simulink model "rx2"  (R2022b)
settings: Solver=FixedStepDiscrete  StartTime=0.0  StopTime=3.3E6  FixedStep=1  RelTol=1e-3  EnableMultiTasking=on
model workspace (MAT data in the model file):
  mwTaskManagerKernelLatency = 0
undefined symbols (not defined in the file or in its folder): Add, jsin, magnitude, rom_pilot_conj_tt, Shift
libraries: hdlsllib x3231, whdlutilities x525, simulink x260, whdlmod x112, whdledac x26, dsphdlmathfun2 x24, commchan3 x1
(part 46 of 59)

== system rx2/demode1/chan_est1/Subsystem/HDL_DUT6/delta_estimator/iteration_estimation/register ==
  data_in : Inport
  valid_in : Inport  Port=2
  to_0 : Inport  Port=3
  Constant : Constant  OutDataTypeStr=fixdt(0,2,0)
  Ground : Ground
  Logical Operator : Logic  Operator=NOT  AllPortsSameDT=off  OutDataTypeStr=boolean
  Simple Dual Port RAM : hdlsllib/HDL RAMs/Simple Dual Port RAM  ram_size=2
  Switch : Switch  Criteria=u2 ~= 0  SaturateOnIntegerOverflow=off  InputSameDT=off
  data_out : Outport
  wires:
  data_in/1 -> Switch/1
  Simple Dual Port RAM/1 -> data_out/1
  Constant/1 -> Simple Dual Port RAM/4, Simple Dual Port RAM/2
  valid_in/1 -> Simple Dual Port RAM/3
  to_0/1 -> Logical Operator/1
  Logical Operator/1 -> Switch/2
  Ground/1 -> Switch/3
  Switch/1 -> Simple Dual Port RAM/1

== system rx2/demode1/chan_est1/Subsystem/HDL_DUT6/delta_estimator/iteration_estimation1/register ==
  data_in : Inport
  valid_in : Inport  Port=2
  to_0 : Inport  Port=3
  Constant : Constant  OutDataTypeStr=fixdt(0,2,0)
  Ground : Ground
  Logical Operator : Logic  Operator=NOT  AllPortsSameDT=off  OutDataTypeStr=boolean
  Simple Dual Port RAM : hdlsllib/HDL RAMs/Simple Dual Port RAM  ram_size=2
  Switch : Switch  Criteria=u2 ~= 0  SaturateOnIntegerOverflow=off  InputSameDT=off
  data_out : Outport
  wires:
  Switch/1 -> Simple Dual Port RAM/1
  Ground/1 -> Switch/3
  Logical Operator/1 -> Switch/2
  to_0/1 -> Logical Operator/1
  valid_in/1 -> Simple Dual Port RAM/3
  Constant/1 -> Simple Dual Port RAM/2, Simple Dual Port RAM/4
  Simple Dual Port RAM/1 -> data_out/1
  data_in/1 -> Switch/1

== system rx2/demode1/chan_est1/Subsystem/HDL_DUT7/delta_estimator/iteration_estimation/register ==
  data_in : Inport
  valid_in : Inport  Port=2
  to_0 : Inport  Port=3
  Constant : Constant  OutDataTypeStr=fixdt(0,2,0)
  Ground : Ground
  Logical Operator : Logic  Operator=NOT  AllPortsSameDT=off  OutDataTypeStr=boolean
  Simple Dual Port RAM : hdlsllib/HDL RAMs/Simple Dual Port RAM  ram_size=2
  Switch : Switch  Criteria=u2 ~= 0  SaturateOnIntegerOverflow=off  InputSameDT=off
  data_out : Outport
  wires:
  data_in/1 -> Switch/1
  Simple Dual Port RAM/1 -> data_out/1
  Constant/1 -> Simple Dual Port RAM/4, Simple Dual Port RAM/2
  valid_in/1 -> Simple Dual Port RAM/3
  to_0/1 -> Logical Operator/1
  Logical Operator/1 -> Switch/2
  Ground/1 -> Switch/3
  Switch/1 -> Simple Dual Port RAM/1

== system rx2/demode1/chan_est1/Subsystem/HDL_DUT7/delta_estimator/iteration_estimation1/register ==
  data_in : Inport
  valid_in : Inport  Port=2
  to_0 : Inport  Port=3
  Constant : Constant  OutDataTypeStr=fixdt(0,2,0)
  Ground : Ground
  Logical Operator : Logic  Operator=NOT  AllPortsSameDT=off  OutDataTypeStr=boolean
  Simple Dual Port RAM : hdlsllib/HDL RAMs/Simple Dual Port RAM  ram_size=2
  Switch : Switch  Criteria=u2 ~= 0  SaturateOnIntegerOverflow=off  InputSameDT=off
  data_out : Outport
  wires:
  Switch/1 -> Simple Dual Port RAM/1
  Ground/1 -> Switch/3
  Logical Operator/1 -> Switch/2
  to_0/1 -> Logical Operator/1
  valid_in/1 -> Simple Dual Port RAM/3
  Constant/1 -> Simple Dual Port RAM/2, Simple Dual Port RAM/4
  Simple Dual Port RAM/1 -> data_out/1
  data_in/1 -> Switch/1

== system rx2/process1/decoder/p-p/Subsystem2/Subsystem/Subsystem1/Subsystem ==
  data1 : Inport  OutDataTypeStr=data_type
  wr_addr : Inport  Port=2
  wr_en1 : Inport  Port=3
  rd_addr : Inport  Port=4
  Mux : Mux  Inputs=2
  Selector : Selector  InputPortWidth=8  IndexOptions=Index vector (dialog)  Indices=[1:4]  OutputSizes=1
  Selector1 : Selector  InputPortWidth=8  IndexOptions=Index vector (dialog)  Indices=[5:8]  OutputSizes=1
  Subsystem1 : Subsystem
  Subsystem4 : Subsystem
  rd_dout : Outport  PortDimensions=8  VectorParamsAs1DForOutWhenUnconnected=off
  wires:
  wr_addr/1 -> Subsystem1/2(wr_addr1), Subsystem4/2(wr_addr1)
  rd_addr/1 -> Subsystem1/4(rd_addr1), Subsystem4/4(rd_addr1)
  wr_en1/1 -> Subsystem1/3(wr_en2), Subsystem4/3(wr_en2)
  Mux/1 -> rd_dout/1
  Subsystem4/1(rd_dout1) -> Mux/1
  Subsystem1/1(rd_dout1) -> Mux/2
  data1/1 -> Selector1/1, Selector/1
  Selector/1 -> Subsystem4/1(data2)
  Selector1/1 -> Subsystem1/1(data2)

== system rx2/process1/decoder/p-p/Subsystem2/Subsystem/Subsystem1/Subsystem1 ==
  data1 : Inport  OutDataTypeStr=data_type
  wr_addr : Inport  Port=2
  wr_en1 : Inport  Port=3
  rd_addr : Inport  Port=4
  Mux : Mux  Inputs=2
  Selector : Selector  InputPortWidth=8  IndexOptions=Index vector (dialog)  Indices=[1:4]  OutputSizes=1
  Selector1 : Selector  InputPortWidth=8  IndexOptions=Index vector (dialog)  Indices=[5:8]  OutputSizes=1
  Subsystem1 : Subsystem
  Subsystem4 : Subsystem
  rd_dout : Outport  PortDimensions=8  VectorParamsAs1DForOutWhenUnconnected=off
  wires:
  Selector1/1 -> Subsystem1/1(data2)
  Selector/1 -> Subsystem4/1(data2)
  data1/1 -> Selector/1, Selector1/1
  Subsystem1/1(rd_dout1) -> Mux/2
  Subsystem4/1(rd_dout1) -> Mux/1
  Mux/1 -> rd_dout/1
  wr_en1/1 -> Subsystem1/3(wr_en2), Subsystem4/3(wr_en2)
  rd_addr/1 -> Subsystem1/4(rd_addr1), Subsystem4/4(rd_addr1)
  wr_addr/1 -> Subsystem1/2(wr_addr1), Subsystem4/2(wr_addr1)

== system rx2/process1/decoder/p-p/Subsystem2/Subsystem/Subsystem2/Subsystem ==
  data1 : Inport  OutDataTypeStr=data_type
  wr_addr : Inport  Port=2
  wr_en1 : Inport  Port=3
  rd_addr : Inport  Port=4
  Mux : Mux  Inputs=2
  Selector : Selector  InputPortWidth=8  IndexOptions=Index vector (dialog)  Indices=[1:4]  OutputSizes=1
  Selector1 : Selector  InputPortWidth=8  IndexOptions=Index vector (dialog)  Indices=[5:8]  OutputSizes=1
  Subsystem1 : Subsystem
  Subsystem4 : Subsystem
  rd_dout : Outport  PortDimensions=8  VectorParamsAs1DForOutWhenUnconnected=off
  wires:
  wr_addr/1 -> Subsystem1/2(wr_addr1), Subsystem4/2(wr_addr1)
  rd_addr/1 -> Subsystem1/4(rd_addr1), Subsystem4/4(rd_addr1)
  wr_en1/1 -> Subsystem1/3(wr_en2), Subsystem4/3(wr_en2)
  Mux/1 -> rd_dout/1
  Subsystem4/1(rd_dout1) -> Mux/1
  Subsystem1/1(rd_dout1) -> Mux/2
  data1/1 -> Selector1/1, Selector/1
  Selector/1 -> Subsystem4/1(data2)
  Selector1/1 -> Subsystem1/1(data2)

== system rx2/process1/decoder/p-p/Subsystem2/Subsystem/Subsystem2/Subsystem1 ==
  data1 : Inport  OutDataTypeStr=data_type
  wr_addr : Inport  Port=2
  wr_en1 : Inport  Port=3
  rd_addr : Inport  Port=4
  Mux : Mux  Inputs=2
  Selector : Selector  InputPortWidth=8  IndexOptions=Index vector (dialog)  Indices=[1:4]  OutputSizes=1
  Selector1 : Selector  InputPortWidth=8  IndexOptions=Index vector (dialog)  Indices=[5:8]  OutputSizes=1
  Subsystem1 : Subsystem
  Subsystem4 : Subsystem
  rd_dout : Outport  PortDimensions=8  VectorParamsAs1DForOutWhenUnconnected=off
  wires:
  Selector1/1 -> Subsystem1/1(data2)
  Selector/1 -> Subsystem4/1(data2)
  data1/1 -> Selector/1, Selector1/1
  Subsystem1/1(rd_dout1) -> Mux/2
  Subsystem4/1(rd_dout1) -> Mux/1
  Mux/1 -> rd_dout/1
  wr_en1/1 -> Subsystem1/3(wr_en2), Subsystem4/3(wr_en2)
  rd_addr/1 -> Subsystem1/4(rd_addr1), Subsystem4/4(rd_addr1)
  wr_addr/1 -> Subsystem1/2(wr_addr1), Subsystem4/2(wr_addr1)

== system rx2/process1/decoder/p-p/Subsystem2/Subsystem1/Subsystem1/Subsystem ==
  data1 : Inport  OutDataTypeStr=data_type
  wr_addr : Inport  Port=2
  wr_en1 : Inport  Port=3
  rd_addr : Inport  Port=4
  Mux : Mux  Inputs=2
  Selector : Selector  InputPortWidth=8  IndexOptions=Index vector (dialog)  Indices=[1:4]  OutputSizes=1
  Selector1 : Selector  InputPortWidth=8  IndexOptions=Index vector (dialog)  Indices=[5:8]  OutputSizes=1
  Subsystem1 : Subsystem
  Subsystem4 : Subsystem
  rd_dout : Outport  PortDimensions=8  VectorParamsAs1DForOutWhenUnconnected=off
  wires:
  wr_addr/1 -> Subsystem1/2(wr_addr1), Subsystem4/2(wr_addr1)
  rd_addr/1 -> Subsystem1/4(rd_addr1), Subsystem4/4(rd_addr1)
  wr_en1/1 -> Subsystem1/3(wr_en2), Subsystem4/3(wr_en2)
  Mux/1 -> rd_dout/1
  Subsystem4/1(rd_dout1) -> Mux/1
  Subsystem1/1(rd_dout1) -> Mux/2
  data1/1 -> Selector1/1, Selector/1
  Selector/1 -> Subsystem4/1(data2)
  Selector1/1 -> Subsystem1/1(data2)

== system rx2/process1/decoder/p-p/Subsystem2/Subsystem1/Subsystem1/Subsystem1 ==
  data1 : Inport  OutDataTypeStr=data_type
  wr_addr : Inport  Port=2
  wr_en1 : Inport  Port=3
  rd_addr : Inport  Port=4
  Mux : Mux  Inputs=2
  Selector : Selector  InputPortWidth=8  IndexOptions=Index vector (dialog)  Indices=[1:4]  OutputSizes=1
  Selector1 : Selector  InputPortWidth=8  IndexOptions=Index vector (dialog)  Indices=[5:8]  OutputSizes=1
  Subsystem1 : Subsystem
  Subsystem4 : Subsystem
  rd_dout : Outport  PortDimensions=8  VectorParamsAs1DForOutWhenUnconnected=off
  wires:
  Selector1/1 -> Subsystem1/1(data2)
  Selector/1 -> Subsystem4/1(data2)
  data1/1 -> Selector/1, Selector1/1
  Subsystem1/1(rd_dout1) -> Mux/2
  Subsystem4/1(rd_dout1) -> Mux/1
  Mux/1 -> rd_dout/1
  wr_en1/1 -> Subsystem1/3(wr_en2), Subsystem4/3(wr_en2)
  rd_addr/1 -> Subsystem1/4(rd_addr1), Subsystem4/4(rd_addr1)
  wr_addr/1 -> Subsystem1/2(wr_addr1), Subsystem4/2(wr_addr1)

== system rx2/process1/decoder/p-p/Subsystem2/Subsystem1/Subsystem2/Subsystem ==
  data1 : Inport  OutDataTypeStr=data_type
  wr_addr : Inport  Port=2
  wr_en1 : Inport  Port=3
  rd_addr : Inport  Port=4
  Mux : Mux  Inputs=2
  Selector : Selector  InputPortWidth=8  IndexOptions=Index vector (dialog)  Indices=[1:4]  OutputSizes=1
  Selector1 : Selector  InputPortWidth=8  IndexOptions=Index vector (dialog)  Indices=[5:8]  OutputSizes=1
  Subsystem1 : Subsystem
  Subsystem4 : Subsystem
  rd_dout : Outport  PortDimensions=8  VectorParamsAs1DForOutWhenUnconnected=off
  wires:
  wr_addr/1 -> Subsystem1/2(wr_addr1), Subsystem4/2(wr_addr1)
  rd_addr/1 -> Subsystem1/4(rd_addr1), Subsystem4/4(rd_addr1)
  wr_en1/1 -> Subsystem1/3(wr_en2), Subsystem4/3(wr_en2)
  Mux/1 -> rd_dout/1
  Subsystem4/1(rd_dout1) -> Mux/1
  Subsystem1/1(rd_dout1) -> Mux/2
  data1/1 -> Selector1/1, Selector/1
  Selector/1 -> Subsystem4/1(data2)
  Selector1/1 -> Subsystem1/1(data2)

== system rx2/process1/decoder/p-p/Subsystem2/Subsystem1/Subsystem2/Subsystem1 ==
  data1 : Inport  OutDataTypeStr=data_type
  wr_addr : Inport  Port=2
  wr_en1 : Inport  Port=3
  rd_addr : Inport  Port=4
  Mux : Mux  Inputs=2
  Selector : Selector  InputPortWidth=8  IndexOptions=Index vector (dialog)  Indices=[1:4]  OutputSizes=1
  Selector1 : Selector  InputPortWidth=8  IndexOptions=Index vector (dialog)  Indices=[5:8]  OutputSizes=1
  Subsystem1 : Subsystem
  Subsystem4 : Subsystem
  rd_dout : Outport  PortDimensions=8  VectorParamsAs1DForOutWhenUnconnected=off
  wires:
  Selector1/1 -> Subsystem1/1(data2)
  Selector/1 -> Subsystem4/1(data2)
  data1/1 -> Selector/1, Selector1/1
  Subsystem1/1(rd_dout1) -> Mux/2
  Subsystem4/1(rd_dout1) -> Mux/1
  Mux/1 -> rd_dout/1
  wr_en1/1 -> Subsystem1/3(wr_en2), Subsystem4/3(wr_en2)
  rd_addr/1 -> Subsystem1/4(rd_addr1), Subsystem4/4(rd_addr1)
  wr_addr/1 -> Subsystem1/2(wr_addr1), Subsystem4/2(wr_addr1)

== system rx2/process10/decoder/p-p/Subsystem2/Subsystem/Subsystem1/Subsystem ==
  data1 : Inport  OutDataTypeStr=data_type
  wr_addr : Inport  Port=2
  wr_en1 : Inport  Port=3
  rd_addr : Inport  Port=4
  Mux : Mux  Inputs=2
  Selector : Selector  InputPortWidth=8  IndexOptions=Index vector (dialog)  Indices=[1:4]  OutputSizes=1
  Selector1 : Selector  InputPortWidth=8  IndexOptions=Index vector (dialog)  Indices=[5:8]  OutputSizes=1
  Subsystem1 : Subsystem
  Subsystem4 : Subsystem
  rd_dout : Outport  PortDimensions=8  VectorParamsAs1DForOutWhenUnconnected=off
  wires:
  wr_addr/1 -> Subsystem1/2(wr_addr1), Subsystem4/2(wr_addr1)
  rd_addr/1 -> Subsystem1/4(rd_addr1), Subsystem4/4(rd_addr1)
  wr_en1/1 -> Subsystem1/3(wr_en2), Subsystem4/3(wr_en2)
  Mux/1 -> rd_dout/1
  Subsystem4/1(rd_dout1) -> Mux/1
  Subsystem1/1(rd_dout1) -> Mux/2
  data1/1 -> Selector1/1, Selector/1
  Selector/1 -> Subsystem4/1(data2)
  Selector1/1 -> Subsystem1/1(data2)

== system rx2/process10/decoder/p-p/Subsystem2/Subsystem/Subsystem1/Subsystem1 ==
  data1 : Inport  OutDataTypeStr=data_type
  wr_addr : Inport  Port=2
  wr_en1 : Inport  Port=3
  rd_addr : Inport  Port=4
  Mux : Mux  Inputs=2
  Selector : Selector  InputPortWidth=8  IndexOptions=Index vector (dialog)  Indices=[1:4]  OutputSizes=1
  Selector1 : Selector  InputPortWidth=8  IndexOptions=Index vector (dialog)  Indices=[5:8]  OutputSizes=1
  Subsystem1 : Subsystem
  Subsystem4 : Subsystem
  rd_dout : Outport  PortDimensions=8  VectorParamsAs1DForOutWhenUnconnected=off
  wires:
  Selector1/1 -> Subsystem1/1(data2)
  Selector/1 -> Subsystem4/1(data2)
  data1/1 -> Selector/1, Selector1/1
  Subsystem1/1(rd_dout1) -> Mux/2
  Subsystem4/1(rd_dout1) -> Mux/1
  Mux/1 -> rd_dout/1
  wr_en1/1 -> Subsystem1/3(wr_en2), Subsystem4/3(wr_en2)
  rd_addr/1 -> Subsystem1/4(rd_addr1), Subsystem4/4(rd_addr1)
  wr_addr/1 -> Subsystem1/2(wr_addr1), Subsystem4/2(wr_addr1)

== system rx2/process10/decoder/p-p/Subsystem2/Subsystem/Subsystem2/Subsystem ==
  data1 : Inport  OutDataTypeStr=data_type
  wr_addr : Inport  Port=2
  wr_en1 : Inport  Port=3
  rd_addr : Inport  Port=4
  Mux : Mux  Inputs=2
  Selector : Selector  InputPortWidth=8  IndexOptions=Index vector (dialog)  Indices=[1:4]  OutputSizes=1
  Selector1 : Selector  InputPortWidth=8  IndexOptions=Index vector (dialog)  Indices=[5:8]  OutputSizes=1
  Subsystem1 : Subsystem
  Subsystem4 : Subsystem
  rd_dout : Outport  PortDimensions=8  VectorParamsAs1DForOutWhenUnconnected=off
  wires:
  wr_addr/1 -> Subsystem1/2(wr_addr1), Subsystem4/2(wr_addr1)
  rd_addr/1 -> Subsystem1/4(rd_addr1), Subsystem4/4(rd_addr1)
  wr_en1/1 -> Subsystem1/3(wr_en2), Subsystem4/3(wr_en2)
  Mux/1 -> rd_dout/1
  Subsystem4/1(rd_dout1) -> Mux/1
  Subsystem1/1(rd_dout1) -> Mux/2
  data1/1 -> Selector1/1, Selector/1
  Selector/1 -> Subsystem4/1(data2)
  Selector1/1 -> Subsystem1/1(data2)

== system rx2/process10/decoder/p-p/Subsystem2/Subsystem/Subsystem2/Subsystem1 ==
  data1 : Inport  OutDataTypeStr=data_type
  wr_addr : Inport  Port=2
  wr_en1 : Inport  Port=3
  rd_addr : Inport  Port=4
  Mux : Mux  Inputs=2
  Selector : Selector  InputPortWidth=8  IndexOptions=Index vector (dialog)  Indices=[1:4]  OutputSizes=1
  Selector1 : Selector  InputPortWidth=8  IndexOptions=Index vector (dialog)  Indices=[5:8]  OutputSizes=1
  Subsystem1 : Subsystem
  Subsystem4 : Subsystem
  rd_dout : Outport  PortDimensions=8  VectorParamsAs1DForOutWhenUnconnected=off
  wires:
  Selector1/1 -> Subsystem1/1(data2)
  Selector/1 -> Subsystem4/1(data2)
  data1/1 -> Selector/1, Selector1/1
  Subsystem1/1(rd_dout1) -> Mux/2
  Subsystem4/1(rd_dout1) -> Mux/1
  Mux/1 -> rd_dout/1
  wr_en1/1 -> Subsystem1/3(wr_en2), Subsystem4/3(wr_en2)
  rd_addr/1 -> Subsystem1/4(rd_addr1), Subsystem4/4(rd_addr1)
  wr_addr/1 -> Subsystem1/2(wr_addr1), Subsystem4/2(wr_addr1)

== system rx2/process10/decoder/p-p/Subsystem2/Subsystem1/Subsystem1/Subsystem ==
  data1 : Inport  OutDataTypeStr=data_type
  wr_addr : Inport  Port=2
  wr_en1 : Inport  Port=3
  rd_addr : Inport  Port=4
  Mux : Mux  Inputs=2
  Selector : Selector  InputPortWidth=8  IndexOptions=Index vector (dialog)  Indices=[1:4]  OutputSizes=1
  Selector1 : Selector  InputPortWidth=8  IndexOptions=Index vector (dialog)  Indices=[5:8]  OutputSizes=1
  Subsystem1 : Subsystem
  Subsystem4 : Subsystem
  rd_dout : Outport  PortDimensions=8  VectorParamsAs1DForOutWhenUnconnected=off
  wires:
  wr_addr/1 -> Subsystem1/2(wr_addr1), Subsystem4/2(wr_addr1)
  rd_addr/1 -> Subsystem1/4(rd_addr1), Subsystem4/4(rd_addr1)
  wr_en1/1 -> Subsystem1/3(wr_en2), Subsystem4/3(wr_en2)
  Mux/1 -> rd_dout/1
  Subsystem4/1(rd_dout1) -> Mux/1
  Subsystem1/1(rd_dout1) -> Mux/2
  data1/1 -> Selector1/1, Selector/1
  Selector/1 -> Subsystem4/1(data2)
  Selector1/1 -> Subsystem1/1(data2)

== system rx2/process10/decoder/p-p/Subsystem2/Subsystem1/Subsystem1/Subsystem1 ==
  data1 : Inport  OutDataTypeStr=data_type
  wr_addr : Inport  Port=2
  wr_en1 : Inport  Port=3
  rd_addr : Inport  Port=4
  Mux : Mux  Inputs=2
  Selector : Selector  InputPortWidth=8  IndexOptions=Index vector (dialog)  Indices=[1:4]  OutputSizes=1
  Selector1 : Selector  InputPortWidth=8  IndexOptions=Index vector (dialog)  Indices=[5:8]  OutputSizes=1
  Subsystem1 : Subsystem
  Subsystem4 : Subsystem
  rd_dout : Outport  PortDimensions=8  VectorParamsAs1DForOutWhenUnconnected=off
  wires:
  Selector1/1 -> Subsystem1/1(data2)
  Selector/1 -> Subsystem4/1(data2)
  data1/1 -> Selector/1, Selector1/1
  Subsystem1/1(rd_dout1) -> Mux/2
  Subsystem4/1(rd_dout1) -> Mux/1
  Mux/1 -> rd_dout/1
  wr_en1/1 -> Subsystem1/3(wr_en2), Subsystem4/3(wr_en2)
  rd_addr/1 -> Subsystem1/4(rd_addr1), Subsystem4/4(rd_addr1)
  wr_addr/1 -> Subsystem1/2(wr_addr1), Subsystem4/2(wr_addr1)

== system rx2/process10/decoder/p-p/Subsystem2/Subsystem1/Subsystem2/Subsystem ==
  data1 : Inport  OutDataTypeStr=data_type
  wr_addr : Inport  Port=2
  wr_en1 : Inport  Port=3
  rd_addr : Inport  Port=4
  Mux : Mux  Inputs=2
  Selector : Selector  InputPortWidth=8  IndexOptions=Index vector (dialog)  Indices=[1:4]  OutputSizes=1
  Selector1 : Selector  InputPortWidth=8  IndexOptions=Index vector (dialog)  Indices=[5:8]  OutputSizes=1
  Subsystem1 : Subsystem
  Subsystem4 : Subsystem
  rd_dout : Outport  PortDimensions=8  VectorParamsAs1DForOutWhenUnconnected=off
  wires:
  wr_addr/1 -> Subsystem1/2(wr_addr1), Subsystem4/2(wr_addr1)
  rd_addr/1 -> Subsystem1/4(rd_addr1), Subsystem4/4(rd_addr1)
  wr_en1/1 -> Subsystem1/3(wr_en2), Subsystem4/3(wr_en2)
  Mux/1 -> rd_dout/1
  Subsystem4/1(rd_dout1) -> Mux/1
  Subsystem1/1(rd_dout1) -> Mux/2
  data1/1 -> Selector1/1, Selector/1
  Selector/1 -> Subsystem4/1(data2)
  Selector1/1 -> Subsystem1/1(data2)

== system rx2/process10/decoder/p-p/Subsystem2/Subsystem1/Subsystem2/Subsystem1 ==
  data1 : Inport  OutDataTypeStr=data_type
  wr_addr : Inport  Port=2
  wr_en1 : Inport  Port=3
  rd_addr : Inport  Port=4
  Mux : Mux  Inputs=2
  Selector : Selector  InputPortWidth=8  IndexOptions=Index vector (dialog)  Indices=[1:4]  OutputSizes=1
  Selector1 : Selector  InputPortWidth=8  IndexOptions=Index vector (dialog)  Indices=[5:8]  OutputSizes=1
  Subsystem1 : Subsystem
  Subsystem4 : Subsystem
  rd_dout : Outport  PortDimensions=8  VectorParamsAs1DForOutWhenUnconnected=off
  wires:
  Selector1/1 -> Subsystem1/1(data2)
  Selector/1 -> Subsystem4/1(data2)
  data1/1 -> Selector/1, Selector1/1
  Subsystem1/1(rd_dout1) -> Mux/2
  Subsystem4/1(rd_dout1) -> Mux/1
  Mux/1 -> rd_dout/1
  wr_en1/1 -> Subsystem1/3(wr_en2), Subsystem4/3(wr_en2)
  rd_addr/1 -> Subsystem1/4(rd_addr1), Subsystem4/4(rd_addr1)
  wr_addr/1 -> Subsystem1/2(wr_addr1), Subsystem4/2(wr_addr1)

== system rx2/process11/decoder/p-p/Subsystem2/Subsystem/Subsystem1/Subsystem ==
  data1 : Inport  OutDataTypeStr=data_type
  wr_addr : Inport  Port=2
  wr_en1 : Inport  Port=3
  rd_addr : Inport  Port=4
  Mux : Mux  Inputs=2
  Selector : Selector  InputPortWidth=8  IndexOptions=Index vector (dialog)  Indices=[1:4]  OutputSizes=1
  Selector1 : Selector  InputPortWidth=8  IndexOptions=Index vector (dialog)  Indices=[5:8]  OutputSizes=1
  Subsystem1 : Subsystem
  Subsystem4 : Subsystem
  rd_dout : Outport  PortDimensions=8  VectorParamsAs1DForOutWhenUnconnected=off
  wires:
  Selector1/1 -> Subsystem1/1(data2)
  Selector/1 -> Subsystem4/1(data2)
  data1/1 -> Selector/1, Selector1/1
  Subsystem1/1(rd_dout1) -> Mux/2
  Subsystem4/1(rd_dout1) -> Mux/1
  Mux/1 -> rd_dout/1
  wr_en1/1 -> Subsystem4/3(wr_en2), Subsystem1/3(wr_en2)
  rd_addr/1 -> Subsystem4/4(rd_addr1), Subsystem1/4(rd_addr1)
  wr_addr/1 -> Subsystem4/2(wr_addr1), Subsystem1/2(wr_addr1)

== system rx2/process11/decoder/p-p/Subsystem2/Subsystem/Subsystem1/Subsystem1 ==
  data1 : Inport  OutDataTypeStr=data_type
  wr_addr : Inport  Port=2
  wr_en1 : Inport  Port=3
  rd_addr : Inport  Port=4
  Mux : Mux  Inputs=2
  Selector : Selector  InputPortWidth=8  IndexOptions=Index vector (dialog)  Indices=[1:4]  OutputSizes=1
  Selector1 : Selector  InputPortWidth=8  IndexOptions=Index vector (dialog)  Indices=[5:8]  OutputSizes=1
  Subsystem1 : Subsystem
  Subsystem4 : Subsystem
  rd_dout : Outport  PortDimensions=8  VectorParamsAs1DForOutWhenUnconnected=off
  wires:
  wr_addr/1 -> Subsystem4/2(wr_addr1), Subsystem1/2(wr_addr1)
  rd_addr/1 -> Subsystem4/4(rd_addr1), Subsystem1/4(rd_addr1)
  wr_en1/1 -> Subsystem4/3(wr_en2), Subsystem1/3(wr_en2)
  Mux/1 -> rd_dout/1
  Subsystem4/1(rd_dout1) -> Mux/1
  Subsystem1/1(rd_dout1) -> Mux/2
  data1/1 -> Selector1/1, Selector/1
  Selector/1 -> Subsystem4/1(data2)
  Selector1/1 -> Subsystem1/1(data2)

== system rx2/process11/decoder/p-p/Subsystem2/Subsystem/Subsystem2/Subsystem ==
  data1 : Inport  OutDataTypeStr=data_type
  wr_addr : Inport  Port=2
  wr_en1 : Inport  Port=3
  rd_addr : Inport  Port=4
  Mux : Mux  Inputs=2
  Selector : Selector  InputPortWidth=8  IndexOptions=Index vector (dialog)  Indices=[1:4]  OutputSizes=1
  Selector1 : Selector  InputPortWidth=8  IndexOptions=Index vector (dialog)  Indices=[5:8]  OutputSizes=1
  Subsystem1 : Subsystem
  Subsystem4 : Subsystem
  rd_dout : Outport  PortDimensions=8  VectorParamsAs1DForOutWhenUnconnected=off
  wires:
  Selector1/1 -> Subsystem1/1(data2)
  Selector/1 -> Subsystem4/1(data2)
  data1/1 -> Selector/1, Selector1/1
  Subsystem1/1(rd_dout1) -> Mux/2
  Subsystem4/1(rd_dout1) -> Mux/1
  Mux/1 -> rd_dout/1
  wr_en1/1 -> Subsystem4/3(wr_en2), Subsystem1/3(wr_en2)
  rd_addr/1 -> Subsystem4/4(rd_addr1), Subsystem1/4(rd_addr1)
  wr_addr/1 -> Subsystem4/2(wr_addr1), Subsystem1/2(wr_addr1)

== system rx2/process11/decoder/p-p/Subsystem2/Subsystem/Subsystem2/Subsystem1 ==
  data1 : Inport  OutDataTypeStr=data_type
  wr_addr : Inport  Port=2
  wr_en1 : Inport  Port=3
  rd_addr : Inport  Port=4
  Mux : Mux  Inputs=2
  Selector : Selector  InputPortWidth=8  IndexOptions=Index vector (dialog)  Indices=[1:4]  OutputSizes=1
  Selector1 : Selector  InputPortWidth=8  IndexOptions=Index vector (dialog)  Indices=[5:8]  OutputSizes=1
  Subsystem1 : Subsystem
  Subsystem4 : Subsystem
  rd_dout : Outport  PortDimensions=8  VectorParamsAs1DForOutWhenUnconnected=off
  wires:
  wr_addr/1 -> Subsystem4/2(wr_addr1), Subsystem1/2(wr_addr1)
  rd_addr/1 -> Subsystem4/4(rd_addr1), Subsystem1/4(rd_addr1)
  wr_en1/1 -> Subsystem4/3(wr_en2), Subsystem1/3(wr_en2)
  Mux/1 -> rd_dout/1
  Subsystem4/1(rd_dout1) -> Mux/1
  Subsystem1/1(rd_dout1) -> Mux/2
  data1/1 -> Selector1/1, Selector/1
  Selector/1 -> Subsystem4/1(data2)
  Selector1/1 -> Subsystem1/1(data2)

== system rx2/process11/decoder/p-p/Subsystem2/Subsystem1/Subsystem1/Subsystem ==
  data1 : Inport  OutDataTypeStr=data_type
  wr_addr : Inport  Port=2
  wr_en1 : Inport  Port=3
  rd_addr : Inport  Port=4
  Mux : Mux  Inputs=2
  Selector : Selector  InputPortWidth=8  IndexOptions=Index vector (dialog)  Indices=[1:4]  OutputSizes=1
  Selector1 : Selector  InputPortWidth=8  IndexOptions=Index vector (dialog)  Indices=[5:8]  OutputSizes=1
  Subsystem1 : Subsystem
  Subsystem4 : Subsystem
  rd_dout : Outport  PortDimensions=8  VectorParamsAs1DForOutWhenUnconnected=off
  wires:
  Selector1/1 -> Subsystem1/1(data2)
  Selector/1 -> Subsystem4/1(data2)
  data1/1 -> Selector/1, Selector1/1
  Subsystem1/1(rd_dout1) -> Mux/2
  Subsystem4/1(rd_dout1) -> Mux/1
  Mux/1 -> rd_dout/1
  wr_en1/1 -> Subsystem4/3(wr_en2), Subsystem1/3(wr_en2)
  rd_addr/1 -> Subsystem4/4(rd_addr1), Subsystem1/4(rd_addr1)
  wr_addr/1 -> Subsystem4/2(wr_addr1), Subsystem1/2(wr_addr1)

== system rx2/process11/decoder/p-p/Subsystem2/Subsystem1/Subsystem1/Subsystem1 ==
  data1 : Inport  OutDataTypeStr=data_type
  wr_addr : Inport  Port=2
  wr_en1 : Inport  Port=3
  rd_addr : Inport  Port=4
  Mux : Mux  Inputs=2
  Selector : Selector  InputPortWidth=8  IndexOptions=Index vector (dialog)  Indices=[1:4]  OutputSizes=1
  Selector1 : Selector  InputPortWidth=8  IndexOptions=Index vector (dialog)  Indices=[5:8]  OutputSizes=1
  Subsystem1 : Subsystem
  Subsystem4 : Subsystem
  rd_dout : Outport  PortDimensions=8  VectorParamsAs1DForOutWhenUnconnected=off
  wires:
  wr_addr/1 -> Subsystem4/2(wr_addr1), Subsystem1/2(wr_addr1)
  rd_addr/1 -> Subsystem4/4(rd_addr1), Subsystem1/4(rd_addr1)
  wr_en1/1 -> Subsystem4/3(wr_en2), Subsystem1/3(wr_en2)
  Mux/1 -> rd_dout/1
  Subsystem4/1(rd_dout1) -> Mux/1
  Subsystem1/1(rd_dout1) -> Mux/2
  data1/1 -> Selector1/1, Selector/1
  Selector/1 -> Subsystem4/1(data2)
  Selector1/1 -> Subsystem1/1(data2)

== system rx2/process11/decoder/p-p/Subsystem2/Subsystem1/Subsystem2/Subsystem ==
  data1 : Inport  OutDataTypeStr=data_type
  wr_addr : Inport  Port=2
  wr_en1 : Inport  Port=3
  rd_addr : Inport  Port=4
  Mux : Mux  Inputs=2
  Selector : Selector  InputPortWidth=8  IndexOptions=Index vector (dialog)  Indices=[1:4]  OutputSizes=1
  Selector1 : Selector  InputPortWidth=8  IndexOptions=Index vector (dialog)  Indices=[5:8]  OutputSizes=1
  Subsystem1 : Subsystem
  Subsystem4 : Subsystem
  rd_dout : Outport  PortDimensions=8  VectorParamsAs1DForOutWhenUnconnected=off
  wires:
  Selector1/1 -> Subsystem1/1(data2)
  Selector/1 -> Subsystem4/1(data2)
  data1/1 -> Selector/1, Selector1/1
  Subsystem1/1(rd_dout1) -> Mux/2
  Subsystem4/1(rd_dout1) -> Mux/1
  Mux/1 -> rd_dout/1
  wr_en1/1 -> Subsystem4/3(wr_en2), Subsystem1/3(wr_en2)
  rd_addr/1 -> Subsystem4/4(rd_addr1), Subsystem1/4(rd_addr1)
  wr_addr/1 -> Subsystem4/2(wr_addr1), Subsystem1/2(wr_addr1)

== system rx2/process11/decoder/p-p/Subsystem2/Subsystem1/Subsystem2/Subsystem1 ==
  data1 : Inport  OutDataTypeStr=data_type
  wr_addr : Inport  Port=2
  wr_en1 : Inport  Port=3
  rd_addr : Inport  Port=4
  Mux : Mux  Inputs=2
  Selector : Selector  InputPortWidth=8  IndexOptions=Index vector (dialog)  Indices=[1:4]  OutputSizes=1
  Selector1 : Selector  InputPortWidth=8  IndexOptions=Index vector (dialog)  Indices=[5:8]  OutputSizes=1
  Subsystem1 : Subsystem
  Subsystem4 : Subsystem
  rd_dout : Outport  PortDimensions=8  VectorParamsAs1DForOutWhenUnconnected=off
  wires:
  wr_addr/1 -> Subsystem4/2(wr_addr1), Subsystem1/2(wr_addr1)
  rd_addr/1 -> Subsystem4/4(rd_addr1), Subsystem1/4(rd_addr1)
  wr_en1/1 -> Subsystem4/3(wr_en2), Subsystem1/3(wr_en2)
  Mux/1 -> rd_dout/1
  Subsystem4/1(rd_dout1) -> Mux/1
  Subsystem1/1(rd_dout1) -> Mux/2
  data1/1 -> Selector1/1, Selector/1
  Selector/1 -> Subsystem4/1(data2)
  Selector1/1 -> Subsystem1/1(data2)

== system rx2/process12/decoder/p-p/Subsystem2/Subsystem/Subsystem1/Subsystem ==
  data1 : Inport  OutDataTypeStr=data_type
  wr_addr : Inport  Port=2
  wr_en1 : Inport  Port=3
  rd_addr : Inport  Port=4
  Mux : Mux  Inputs=2
  Selector : Selector  InputPortWidth=8  IndexOptions=Index vector (dialog)  Indices=[1:4]  OutputSizes=1
  Selector1 : Selector  InputPortWidth=8  IndexOptions=Index vector (dialog)  Indices=[5:8]  OutputSizes=1
  Subsystem1 : Subsystem
  Subsystem4 : Subsystem
  rd_dout : Outport  PortDimensions=8  VectorParamsAs1DForOutWhenUnconnected=off
  wires:
  wr_addr/1 -> Subsystem1/2(wr_addr1), Subsystem4/2(wr_addr1)
  rd_addr/1 -> Subsystem1/4(rd_addr1), Subsystem4/4(rd_addr1)
  wr_en1/1 -> Subsystem1/3(wr_en2), Subsystem4/3(wr_en2)
  Mux/1 -> rd_dout/1
  Subsystem4/1(rd_dout1) -> Mux/1
  Subsystem1/1(rd_dout1) -> Mux/2
  data1/1 -> Selector1/1, Selector/1
  Selector/1 -> Subsystem4/1(data2)
  Selector1/1 -> Subsystem1/1(data2)

== system rx2/process12/decoder/p-p/Subsystem2/Subsystem/Subsystem1/Subsystem1 ==
  data1 : Inport  OutDataTypeStr=data_type
  wr_addr : Inport  Port=2
  wr_en1 : Inport  Port=3
  rd_addr : Inport  Port=4
  Mux : Mux  Inputs=2
  Selector : Selector  InputPortWidth=8  IndexOptions=Index vector (dialog)  Indices=[1:4]  OutputSizes=1
  Selector1 : Selector  InputPortWidth=8  IndexOptions=Index vector (dialog)  Indices=[5:8]  OutputSizes=1
  Subsystem1 : Subsystem
  Subsystem4 : Subsystem
  rd_dout : Outport  PortDimensions=8  VectorParamsAs1DForOutWhenUnconnected=off
  wires:
  Selector1/1 -> Subsystem1/1(data2)
  Selector/1 -> Subsystem4/1(data2)
  data1/1 -> Selector/1, Selector1/1
  Subsystem1/1(rd_dout1) -> Mux/2
  Subsystem4/1(rd_dout1) -> Mux/1
  Mux/1 -> rd_dout/1
  wr_en1/1 -> Subsystem1/3(wr_en2), Subsystem4/3(wr_en2)
  rd_addr/1 -> Subsystem1/4(rd_addr1), Subsystem4/4(rd_addr1)
  wr_addr/1 -> Subsystem1/2(wr_addr1), Subsystem4/2(wr_addr1)

== system rx2/process12/decoder/p-p/Subsystem2/Subsystem/Subsystem2/Subsystem ==
  data1 : Inport  OutDataTypeStr=data_type
  wr_addr : Inport  Port=2
  wr_en1 : Inport  Port=3
  rd_addr : Inport  Port=4
  Mux : Mux  Inputs=2
  Selector : Selector  InputPortWidth=8  IndexOptions=Index vector (dialog)  Indices=[1:4]  OutputSizes=1
  Selector1 : Selector  InputPortWidth=8  IndexOptions=Index vector (dialog)  Indices=[5:8]  OutputSizes=1
  Subsystem1 : Subsystem
  Subsystem4 : Subsystem
  rd_dout : Outport  PortDimensions=8  VectorParamsAs1DForOutWhenUnconnected=off
  wires:
  wr_addr/1 -> Subsystem1/2(wr_addr1), Subsystem4/2(wr_addr1)
  rd_addr/1 -> Subsystem1/4(rd_addr1), Subsystem4/4(rd_addr1)
  wr_en1/1 -> Subsystem1/3(wr_en2), Subsystem4/3(wr_en2)
  Mux/1 -> rd_dout/1
  Subsystem4/1(rd_dout1) -> Mux/1
  Subsystem1/1(rd_dout1) -> Mux/2
  data1/1 -> Selector1/1, Selector/1
  Selector/1 -> Subsystem4/1(data2)
  Selector1/1 -> Subsystem1/1(data2)

== system rx2/process12/decoder/p-p/Subsystem2/Subsystem/Subsystem2/Subsystem1 ==
  data1 : Inport  OutDataTypeStr=data_type
  wr_addr : Inport  Port=2
  wr_en1 : Inport  Port=3
  rd_addr : Inport  Port=4
  Mux : Mux  Inputs=2
  Selector : Selector  InputPortWidth=8  IndexOptions=Index vector (dialog)  Indices=[1:4]  OutputSizes=1
  Selector1 : Selector  InputPortWidth=8  IndexOptions=Index vector (dialog)  Indices=[5:8]  OutputSizes=1
  Subsystem1 : Subsystem
  Subsystem4 : Subsystem
  rd_dout : Outport  PortDimensions=8  VectorParamsAs1DForOutWhenUnconnected=off
  wires:
  Selector1/1 -> Subsystem1/1(data2)
  Selector/1 -> Subsystem4/1(data2)
  data1/1 -> Selector/1, Selector1/1
  Subsystem1/1(rd_dout1) -> Mux/2
  Subsystem4/1(rd_dout1) -> Mux/1
  Mux/1 -> rd_dout/1
  wr_en1/1 -> Subsystem1/3(wr_en2), Subsystem4/3(wr_en2)
  rd_addr/1 -> Subsystem1/4(rd_addr1), Subsystem4/4(rd_addr1)
  wr_addr/1 -> Subsystem1/2(wr_addr1), Subsystem4/2(wr_addr1)

== system rx2/process12/decoder/p-p/Subsystem2/Subsystem1/Subsystem1/Subsystem ==
  data1 : Inport  OutDataTypeStr=data_type
  wr_addr : Inport  Port=2
  wr_en1 : Inport  Port=3
  rd_addr : Inport  Port=4
  Mux : Mux  Inputs=2
  Selector : Selector  InputPortWidth=8  IndexOptions=Index vector (dialog)  Indices=[1:4]  OutputSizes=1
  Selector1 : Selector  InputPortWidth=8  IndexOptions=Index vector (dialog)  Indices=[5:8]  OutputSizes=1
  Subsystem1 : Subsystem
  Subsystem4 : Subsystem
  rd_dout : Outport  PortDimensions=8  VectorParamsAs1DForOutWhenUnconnected=off
  wires:
  wr_addr/1 -> Subsystem1/2(wr_addr1), Subsystem4/2(wr_addr1)
  rd_addr/1 -> Subsystem1/4(rd_addr1), Subsystem4/4(rd_addr1)
  wr_en1/1 -> Subsystem1/3(wr_en2), Subsystem4/3(wr_en2)
  Mux/1 -> rd_dout/1
  Subsystem4/1(rd_dout1) -> Mux/1
  Subsystem1/1(rd_dout1) -> Mux/2
  data1/1 -> Selector1/1, Selector/1
  Selector/1 -> Subsystem4/1(data2)
  Selector1/1 -> Subsystem1/1(data2)

== system rx2/process12/decoder/p-p/Subsystem2/Subsystem1/Subsystem1/Subsystem1 ==
  data1 : Inport  OutDataTypeStr=data_type
  wr_addr : Inport  Port=2
  wr_en1 : Inport  Port=3
  rd_addr : Inport  Port=4
  Mux : Mux  Inputs=2
  Selector : Selector  InputPortWidth=8  IndexOptions=Index vector (dialog)  Indices=[1:4]  OutputSizes=1
  Selector1 : Selector  InputPortWidth=8  IndexOptions=Index vector (dialog)  Indices=[5:8]  OutputSizes=1
  Subsystem1 : Subsystem
  Subsystem4 : Subsystem
  rd_dout : Outport  PortDimensions=8  VectorParamsAs1DForOutWhenUnconnected=off
  wires:
  Selector1/1 -> Subsystem1/1(data2)
  Selector/1 -> Subsystem4/1(data2)
  data1/1 -> Selector/1, Selector1/1
  Subsystem1/1(rd_dout1) -> Mux/2
  Subsystem4/1(rd_dout1) -> Mux/1
  Mux/1 -> rd_dout/1
  wr_en1/1 -> Subsystem1/3(wr_en2), Subsystem4/3(wr_en2)
  rd_addr/1 -> Subsystem1/4(rd_addr1), Subsystem4/4(rd_addr1)
  wr_addr/1 -> Subsystem1/2(wr_addr1), Subsystem4/2(wr_addr1)

== system rx2/process12/decoder/p-p/Subsystem2/Subsystem1/Subsystem2/Subsystem ==
  data1 : Inport  OutDataTypeStr=data_type
  wr_addr : Inport  Port=2
  wr_en1 : Inport  Port=3
  rd_addr : Inport  Port=4
  Mux : Mux  Inputs=2
  Selector : Selector  InputPortWidth=8  IndexOptions=Index vector (dialog)  Indices=[1:4]  OutputSizes=1
  Selector1 : Selector  InputPortWidth=8  IndexOptions=Index vector (dialog)  Indices=[5:8]  OutputSizes=1
  Subsystem1 : Subsystem
  Subsystem4 : Subsystem
  rd_dout : Outport  PortDimensions=8  VectorParamsAs1DForOutWhenUnconnected=off
  wires:
  wr_addr/1 -> Subsystem1/2(wr_addr1), Subsystem4/2(wr_addr1)
  rd_addr/1 -> Subsystem1/4(rd_addr1), Subsystem4/4(rd_addr1)
  wr_en1/1 -> Subsystem1/3(wr_en2), Subsystem4/3(wr_en2)
  Mux/1 -> rd_dout/1
  Subsystem4/1(rd_dout1) -> Mux/1
  Subsystem1/1(rd_dout1) -> Mux/2
  data1/1 -> Selector1/1, Selector/1
  Selector/1 -> Subsystem4/1(data2)
  Selector1/1 -> Subsystem1/1(data2)

== system rx2/process12/decoder/p-p/Subsystem2/Subsystem1/Subsystem2/Subsystem1 ==
  data1 : Inport  OutDataTypeStr=data_type
  wr_addr : Inport  Port=2
  wr_en1 : Inport  Port=3
  rd_addr : Inport  Port=4
  Mux : Mux  Inputs=2
  Selector : Selector  InputPortWidth=8  IndexOptions=Index vector (dialog)  Indices=[1:4]  OutputSizes=1
  Selector1 : Selector  InputPortWidth=8  IndexOptions=Index vector (dialog)  Indices=[5:8]  OutputSizes=1
  Subsystem1 : Subsystem
  Subsystem4 : Subsystem
  rd_dout : Outport  PortDimensions=8  VectorParamsAs1DForOutWhenUnconnected=off
  wires:
  Selector1/1 -> Subsystem1/1(data2)
  Selector/1 -> Subsystem4/1(data2)
  data1/1 -> Selector/1, Selector1/1
  Subsystem1/1(rd_dout1) -> Mux/2
  Subsystem4/1(rd_dout1) -> Mux/1
  Mux/1 -> rd_dout/1
  wr_en1/1 -> Subsystem1/3(wr_en2), Subsystem4/3(wr_en2)
  rd_addr/1 -> Subsystem1/4(rd_addr1), Subsystem4/4(rd_addr1)
  wr_addr/1 -> Subsystem1/2(wr_addr1), Subsystem4/2(wr_addr1)

== system rx2/process13/decoder/p-p/Subsystem2/Subsystem/Subsystem1/Subsystem ==
  data1 : Inport  OutDataTypeStr=data_type
  wr_addr : Inport  Port=2
  wr_en1 : Inport  Port=3
  rd_addr : Inport  Port=4
  Mux : Mux  Inputs=2
  Selector : Selector  InputPortWidth=8  IndexOptions=Index vector (dialog)  Indices=[1:4]  OutputSizes=1
  Selector1 : Selector  InputPortWidth=8  IndexOptions=Index vector (dialog)  Indices=[5:8]  OutputSizes=1
  Subsystem1 : Subsystem
  Subsystem4 : Subsystem
  rd_dout : Outport  PortDimensions=8  VectorParamsAs1DForOutWhenUnconnected=off
  wires:
  Selector1/1 -> Subsystem1/1(data2)
  Selector/1 -> Subsystem4/1(data2)
  data1/1 -> Selector/1, Selector1/1
  Subsystem1/1(rd_dout1) -> Mux/2
  Subsystem4/1(rd_dout1) -> Mux/1
  Mux/1 -> rd_dout/1
  wr_en1/1 -> Subsystem4/3(wr_en2), Subsystem1/3(wr_en2)
  rd_addr/1 -> Subsystem4/4(rd_addr1), Subsystem1/4(rd_addr1)
  wr_addr/1 -> Subsystem4/2(wr_addr1), Subsystem1/2(wr_addr1)

== system rx2/process13/decoder/p-p/Subsystem2/Subsystem/Subsystem1/Subsystem1 ==
  data1 : Inport  OutDataTypeStr=data_type
  wr_addr : Inport  Port=2
  wr_en1 : Inport  Port=3
  rd_addr : Inport  Port=4
  Mux : Mux  Inputs=2
  Selector : Selector  InputPortWidth=8  IndexOptions=Index vector (dialog)  Indices=[1:4]  OutputSizes=1
  Selector1 : Selector  InputPortWidth=8  IndexOptions=Index vector (dialog)  Indices=[5:8]  OutputSizes=1
  Subsystem1 : Subsystem
  Subsystem4 : Subsystem
  rd_dout : Outport  PortDimensions=8  VectorParamsAs1DForOutWhenUnconnected=off
  wires:
  wr_addr/1 -> Subsystem4/2(wr_addr1), Subsystem1/2(wr_addr1)
  rd_addr/1 -> Subsystem4/4(rd_addr1), Subsystem1/4(rd_addr1)
  wr_en1/1 -> Subsystem4/3(wr_en2), Subsystem1/3(wr_en2)
  Mux/1 -> rd_dout/1
  Subsystem4/1(rd_dout1) -> Mux/1
  Subsystem1/1(rd_dout1) -> Mux/2
  data1/1 -> Selector1/1, Selector/1
  Selector/1 -> Subsystem4/1(data2)
  Selector1/1 -> Subsystem1/1(data2)

== system rx2/process13/decoder/p-p/Subsystem2/Subsystem/Subsystem2/Subsystem ==
  data1 : Inport  OutDataTypeStr=data_type
  wr_addr : Inport  Port=2
  wr_en1 : Inport  Port=3
  rd_addr : Inport  Port=4
  Mux : Mux  Inputs=2
  Selector : Selector  InputPortWidth=8  IndexOptions=Index vector (dialog)  Indices=[1:4]  OutputSizes=1
  Selector1 : Selector  InputPortWidth=8  IndexOptions=Index vector (dialog)  Indices=[5:8]  OutputSizes=1
  Subsystem1 : Subsystem
  Subsystem4 : Subsystem
  rd_dout : Outport  PortDimensions=8  VectorParamsAs1DForOutWhenUnconnected=off
  wires:
  Selector1/1 -> Subsystem1/1(data2)
  Selector/1 -> Subsystem4/1(data2)
  data1/1 -> Selector/1, Selector1/1
  Subsystem1/1(rd_dout1) -> Mux/2
  Subsystem4/1(rd_dout1) -> Mux/1
  Mux/1 -> rd_dout/1
  wr_en1/1 -> Subsystem4/3(wr_en2), Subsystem1/3(wr_en2)
  rd_addr/1 -> Subsystem4/4(rd_addr1), Subsystem1/4(rd_addr1)
  wr_addr/1 -> Subsystem4/2(wr_addr1), Subsystem1/2(wr_addr1)

== system rx2/process13/decoder/p-p/Subsystem2/Subsystem/Subsystem2/Subsystem1 ==
  data1 : Inport  OutDataTypeStr=data_type
  wr_addr : Inport  Port=2
  wr_en1 : Inport  Port=3
  rd_addr : Inport  Port=4
  Mux : Mux  Inputs=2
  Selector : Selector  InputPortWidth=8  IndexOptions=Index vector (dialog)  Indices=[1:4]  OutputSizes=1
  Selector1 : Selector  InputPortWidth=8  IndexOptions=Index vector (dialog)  Indices=[5:8]  OutputSizes=1
  Subsystem1 : Subsystem
  Subsystem4 : Subsystem
  rd_dout : Outport  PortDimensions=8  VectorParamsAs1DForOutWhenUnconnected=off
  wires:
  wr_addr/1 -> Subsystem4/2(wr_addr1), Subsystem1/2(wr_addr1)
  rd_addr/1 -> Subsystem4/4(rd_addr1), Subsystem1/4(rd_addr1)
  wr_en1/1 -> Subsystem4/3(wr_en2), Subsystem1/3(wr_en2)
  Mux/1 -> rd_dout/1
  Subsystem4/1(rd_dout1) -> Mux/1
  Subsystem1/1(rd_dout1) -> Mux/2
  data1/1 -> Selector1/1, Selector/1
  Selector/1 -> Subsystem4/1(data2)
  Selector1/1 -> Subsystem1/1(data2)

== system rx2/process13/decoder/p-p/Subsystem2/Subsystem1/Subsystem1/Subsystem ==
  data1 : Inport  OutDataTypeStr=data_type
  wr_addr : Inport  Port=2
  wr_en1 : Inport  Port=3
  rd_addr : Inport  Port=4
  Mux : Mux  Inputs=2
  Selector : Selector  InputPortWidth=8  IndexOptions=Index vector (dialog)  Indices=[1:4]  OutputSizes=1
  Selector1 : Selector  InputPortWidth=8  IndexOptions=Index vector (dialog)  Indices=[5:8]  OutputSizes=1
  Subsystem1 : Subsystem
  Subsystem4 : Subsystem
  rd_dout : Outport  PortDimensions=8  VectorParamsAs1DForOutWhenUnconnected=off
  wires:
  Selector1/1 -> Subsystem1/1(data2)
  Selector/1 -> Subsystem4/1(data2)
  data1/1 -> Selector/1, Selector1/1
  Subsystem1/1(rd_dout1) -> Mux/2
  Subsystem4/1(rd_dout1) -> Mux/1
  Mux/1 -> rd_dout/1
  wr_en1/1 -> Subsystem4/3(wr_en2), Subsystem1/3(wr_en2)
  rd_addr/1 -> Subsystem4/4(rd_addr1), Subsystem1/4(rd_addr1)
  wr_addr/1 -> Subsystem4/2(wr_addr1), Subsystem1/2(wr_addr1)

== system rx2/process13/decoder/p-p/Subsystem2/Subsystem1/Subsystem1/Subsystem1 ==
  data1 : Inport  OutDataTypeStr=data_type
  wr_addr : Inport  Port=2
  wr_en1 : Inport  Port=3
  rd_addr : Inport  Port=4
  Mux : Mux  Inputs=2
  Selector : Selector  InputPortWidth=8  IndexOptions=Index vector (dialog)  Indices=[1:4]  OutputSizes=1
  Selector1 : Selector  InputPortWidth=8  IndexOptions=Index vector (dialog)  Indices=[5:8]  OutputSizes=1
  Subsystem1 : Subsystem
  Subsystem4 : Subsystem
  rd_dout : Outport  PortDimensions=8  VectorParamsAs1DForOutWhenUnconnected=off
  wires:
  wr_addr/1 -> Subsystem4/2(wr_addr1), Subsystem1/2(wr_addr1)
  rd_addr/1 -> Subsystem4/4(rd_addr1), Subsystem1/4(rd_addr1)
  wr_en1/1 -> Subsystem4/3(wr_en2), Subsystem1/3(wr_en2)
  Mux/1 -> rd_dout/1
  Subsystem4/1(rd_dout1) -> Mux/1
  Subsystem1/1(rd_dout1) -> Mux/2
  data1/1 -> Selector1/1, Selector/1
  Selector/1 -> Subsystem4/1(data2)
  Selector1/1 -> Subsystem1/1(data2)

== system rx2/process13/decoder/p-p/Subsystem2/Subsystem1/Subsystem2/Subsystem ==
  data1 : Inport  OutDataTypeStr=data_type
  wr_addr : Inport  Port=2
  wr_en1 : Inport  Port=3
  rd_addr : Inport  Port=4
  Mux : Mux  Inputs=2
  Selector : Selector  InputPortWidth=8  IndexOptions=Index vector (dialog)  Indices=[1:4]  OutputSizes=1
  Selector1 : Selector  InputPortWidth=8  IndexOptions=Index vector (dialog)  Indices=[5:8]  OutputSizes=1
  Subsystem1 : Subsystem
  Subsystem4 : Subsystem
  rd_dout : Outport  PortDimensions=8  VectorParamsAs1DForOutWhenUnconnected=off
  wires:
  Selector1/1 -> Subsystem1/1(data2)
  Selector/1 -> Subsystem4/1(data2)
  data1/1 -> Selector/1, Selector1/1
  Subsystem1/1(rd_dout1) -> Mux/2
  Subsystem4/1(rd_dout1) -> Mux/1
  Mux/1 -> rd_dout/1
  wr_en1/1 -> Subsystem4/3(wr_en2), Subsystem1/3(wr_en2)
  rd_addr/1 -> Subsystem4/4(rd_addr1), Subsystem1/4(rd_addr1)
  wr_addr/1 -> Subsystem4/2(wr_addr1), Subsystem1/2(wr_addr1)

== system rx2/process13/decoder/p-p/Subsystem2/Subsystem1/Subsystem2/Subsystem1 ==
  data1 : Inport  OutDataTypeStr=data_type
  wr_addr : Inport  Port=2
  wr_en1 : Inport  Port=3
  rd_addr : Inport  Port=4
  Mux : Mux  Inputs=2
  Selector : Selector  InputPortWidth=8  IndexOptions=Index vector (dialog)  Indices=[1:4]  OutputSizes=1
  Selector1 : Selector  InputPortWidth=8  IndexOptions=Index vector (dialog)  Indices=[5:8]  OutputSizes=1
  Subsystem1 : Subsystem
  Subsystem4 : Subsystem
  rd_dout : Outport  PortDimensions=8  VectorParamsAs1DForOutWhenUnconnected=off
  wires:
  wr_addr/1 -> Subsystem4/2(wr_addr1), Subsystem1/2(wr_addr1)
  rd_addr/1 -> Subsystem4/4(rd_addr1), Subsystem1/4(rd_addr1)
  wr_en1/1 -> Subsystem4/3(wr_en2), Subsystem1/3(wr_en2)
  Mux/1 -> rd_dout/1
  Subsystem4/1(rd_dout1) -> Mux/1
  Subsystem1/1(rd_dout1) -> Mux/2
  data1/1 -> Selector1/1, Selector/1
  Selector/1 -> Subsystem4/1(data2)
  Selector1/1 -> Subsystem1/1(data2)

== system rx2/process2/decoder/p-p/Subsystem2/Subsystem/Subsystem1/Subsystem ==
  data1 : Inport  OutDataTypeStr=data_type
  wr_addr : Inport  Port=2
  wr_en1 : Inport  Port=3
  rd_addr : Inport  Port=4
  Mux : Mux  Inputs=2
  Selector : Selector  InputPortWidth=8  IndexOptions=Index vector (dialog)  Indices=[1:4]  OutputSizes=1
  Selector1 : Selector  InputPortWidth=8  IndexOptions=Index vector (dialog)  Indices=[5:8]  OutputSizes=1
  Subsystem1 : Subsystem
  Subsystem4 : Subsystem
  rd_dout : Outport  PortDimensions=8  VectorParamsAs1DForOutWhenUnconnected=off
  wires:
  wr_addr/1 -> Subsystem1/2(wr_addr1), Subsystem4/2(wr_addr1)
  rd_addr/1 -> Subsystem1/4(rd_addr1), Subsystem4/4(rd_addr1)
  wr_en1/1 -> Subsystem1/3(wr_en2), Subsystem4/3(wr_en2)
  Mux/1 -> rd_dout/1
  Subsystem4/1(rd_dout1) -> Mux/1
  Subsystem1/1(rd_dout1) -> Mux/2
  data1/1 -> Selector1/1, Selector/1
  Selector/1 -> Subsystem4/1(data2)
  Selector1/1 -> Subsystem1/1(data2)

== system rx2/process2/decoder/p-p/Subsystem2/Subsystem/Subsystem1/Subsystem1 ==
  data1 : Inport  OutDataTypeStr=data_type
  wr_addr : Inport  Port=2
  wr_en1 : Inport  Port=3
  rd_addr : Inport  Port=4
  Mux : Mux  Inputs=2
  Selector : Selector  InputPortWidth=8  IndexOptions=Index vector (dialog)  Indices=[1:4]  OutputSizes=1
  Selector1 : Selector  InputPortWidth=8  IndexOptions=Index vector (dialog)  Indices=[5:8]  OutputSizes=1
  Subsystem1 : Subsystem
  Subsystem4 : Subsystem
  rd_dout : Outport  PortDimensions=8  VectorParamsAs1DForOutWhenUnconnected=off
  wires:
  Selector1/1 -> Subsystem1/1(data2)
  Selector/1 -> Subsystem4/1(data2)
  data1/1 -> Selector/1, Selector1/1
  Subsystem1/1(rd_dout1) -> Mux/2
  Subsystem4/1(rd_dout1) -> Mux/1
  Mux/1 -> rd_dout/1
  wr_en1/1 -> Subsystem1/3(wr_en2), Subsystem4/3(wr_en2)
  rd_addr/1 -> Subsystem1/4(rd_addr1), Subsystem4/4(rd_addr1)
  wr_addr/1 -> Subsystem1/2(wr_addr1), Subsystem4/2(wr_addr1)

== system rx2/process2/decoder/p-p/Subsystem2/Subsystem/Subsystem2/Subsystem ==
  data1 : Inport  OutDataTypeStr=data_type
  wr_addr : Inport  Port=2
  wr_en1 : Inport  Port=3
  rd_addr : Inport  Port=4
  Mux : Mux  Inputs=2
  Selector : Selector  InputPortWidth=8  IndexOptions=Index vector (dialog)  Indices=[1:4]  OutputSizes=1
  Selector1 : Selector  InputPortWidth=8  IndexOptions=Index vector (dialog)  Indices=[5:8]  OutputSizes=1
  Subsystem1 : Subsystem
  Subsystem4 : Subsystem
  rd_dout : Outport  PortDimensions=8  VectorParamsAs1DForOutWhenUnconnected=off
  wires:
  wr_addr/1 -> Subsystem1/2(wr_addr1), Subsystem4/2(wr_addr1)
  rd_addr/1 -> Subsystem1/4(rd_addr1), Subsystem4/4(rd_addr1)
  wr_en1/1 -> Subsystem1/3(wr_en2), Subsystem4/3(wr_en2)
  Mux/1 -> rd_dout/1
  Subsystem4/1(rd_dout1) -> Mux/1
  Subsystem1/1(rd_dout1) -> Mux/2
  data1/1 -> Selector1/1, Selector/1
  Selector/1 -> Subsystem4/1(data2)
  Selector1/1 -> Subsystem1/1(data2)

== system rx2/process2/decoder/p-p/Subsystem2/Subsystem/Subsystem2/Subsystem1 ==
  data1 : Inport  OutDataTypeStr=data_type
  wr_addr : Inport  Port=2
  wr_en1 : Inport  Port=3
  rd_addr : Inport  Port=4
  Mux : Mux  Inputs=2
  Selector : Selector  InputPortWidth=8  IndexOptions=Index vector (dialog)  Indices=[1:4]  OutputSizes=1
  Selector1 : Selector  InputPortWidth=8  IndexOptions=Index vector (dialog)  Indices=[5:8]  OutputSizes=1
  Subsystem1 : Subsystem
  Subsystem4 : Subsystem
  rd_dout : Outport  PortDimensions=8  VectorParamsAs1DForOutWhenUnconnected=off
  wires:
  Selector1/1 -> Subsystem1/1(data2)
  Selector/1 -> Subsystem4/1(data2)
  data1/1 -> Selector/1, Selector1/1
  Subsystem1/1(rd_dout1) -> Mux/2
  Subsystem4/1(rd_dout1) -> Mux/1
  Mux/1 -> rd_dout/1
  wr_en1/1 -> Subsystem1/3(wr_en2), Subsystem4/3(wr_en2)
  rd_addr/1 -> Subsystem1/4(rd_addr1), Subsystem4/4(rd_addr1)
  wr_addr/1 -> Subsystem1/2(wr_addr1), Subsystem4/2(wr_addr1)

== system rx2/process2/decoder/p-p/Subsystem2/Subsystem1/Subsystem1/Subsystem ==
  data1 : Inport  OutDataTypeStr=data_type
  wr_addr : Inport  Port=2
  wr_en1 : Inport  Port=3
  rd_addr : Inport  Port=4
  Mux : Mux  Inputs=2
  Selector : Selector  InputPortWidth=8  IndexOptions=Index vector (dialog)  Indices=[1:4]  OutputSizes=1
  Selector1 : Selector  InputPortWidth=8  IndexOptions=Index vector (dialog)  Indices=[5:8]  OutputSizes=1
  Subsystem1 : Subsystem
  Subsystem4 : Subsystem
  rd_dout : Outport  PortDimensions=8  VectorParamsAs1DForOutWhenUnconnected=off
  wires:
  wr_addr/1 -> Subsystem1/2(wr_addr1), Subsystem4/2(wr_addr1)
  rd_addr/1 -> Subsystem1/4(rd_addr1), Subsystem4/4(rd_addr1)
  wr_en1/1 -> Subsystem1/3(wr_en2), Subsystem4/3(wr_en2)
  Mux/1 -> rd_dout/1
  Subsystem4/1(rd_dout1) -> Mux/1
  Subsystem1/1(rd_dout1) -> Mux/2
  data1/1 -> Selector1/1, Selector/1
  Selector/1 -> Subsystem4/1(data2)
  Selector1/1 -> Subsystem1/1(data2)

== system rx2/process2/decoder/p-p/Subsystem2/Subsystem1/Subsystem1/Subsystem1 ==
  data1 : Inport  OutDataTypeStr=data_type
  wr_addr : Inport  Port=2
  wr_en1 : Inport  Port=3
  rd_addr : Inport  Port=4
  Mux : Mux  Inputs=2
  Selector : Selector  InputPortWidth=8  IndexOptions=Index vector (dialog)  Indices=[1:4]  OutputSizes=1
  Selector1 : Selector  InputPortWidth=8  IndexOptions=Index vector (dialog)  Indices=[5:8]  OutputSizes=1
  Subsystem1 : Subsystem
  Subsystem4 : Subsystem
  rd_dout : Outport  PortDimensions=8  VectorParamsAs1DForOutWhenUnconnected=off
  wires:
  Selector1/1 -> Subsystem1/1(data2)
  Selector/1 -> Subsystem4/1(data2)
  data1/1 -> Selector/1, Selector1/1
  Subsystem1/1(rd_dout1) -> Mux/2
  Subsystem4/1(rd_dout1) -> Mux/1
  Mux/1 -> rd_dout/1
  wr_en1/1 -> Subsystem1/3(wr_en2), Subsystem4/3(wr_en2)
  rd_addr/1 -> Subsystem1/4(rd_addr1), Subsystem4/4(rd_addr1)
  wr_addr/1 -> Subsystem1/2(wr_addr1), Subsystem4/2(wr_addr1)

== system rx2/process2/decoder/p-p/Subsystem2/Subsystem1/Subsystem2/Subsystem ==
  data1 : Inport  OutDataTypeStr=data_type
  wr_addr : Inport  Port=2
  wr_en1 : Inport  Port=3
  rd_addr : Inport  Port=4
  Mux : Mux  Inputs=2
  Selector : Selector  InputPortWidth=8  IndexOptions=Index vector (dialog)  Indices=[1:4]  OutputSizes=1
  Selector1 : Selector  InputPortWidth=8  IndexOptions=Index vector (dialog)  Indices=[5:8]  OutputSizes=1
  Subsystem1 : Subsystem
  Subsystem4 : Subsystem
  rd_dout : Outport  PortDimensions=8  VectorParamsAs1DForOutWhenUnconnected=off
  wires:
  wr_addr/1 -> Subsystem1/2(wr_addr1), Subsystem4/2(wr_addr1)
  rd_addr/1 -> Subsystem1/4(rd_addr1), Subsystem4/4(rd_addr1)
  wr_en1/1 -> Subsystem1/3(wr_en2), Subsystem4/3(wr_en2)
  Mux/1 -> rd_dout/1
  Subsystem4/1(rd_dout1) -> Mux/1
  Subsystem1/1(rd_dout1) -> Mux/2
  data1/1 -> Selector1/1, Selector/1
  Selector/1 -> Subsystem4/1(data2)
  Selector1/1 -> Subsystem1/1(data2)

== system rx2/process2/decoder/p-p/Subsystem2/Subsystem1/Subsystem2/Subsystem1 ==
  data1 : Inport  OutDataTypeStr=data_type
  wr_addr : Inport  Port=2
  wr_en1 : Inport  Port=3
  rd_addr : Inport  Port=4
  Mux : Mux  Inputs=2
  Selector : Selector  InputPortWidth=8  IndexOptions=Index vector (dialog)  Indices=[1:4]  OutputSizes=1
  Selector1 : Selector  InputPortWidth=8  IndexOptions=Index vector (dialog)  Indices=[5:8]  OutputSizes=1
  Subsystem1 : Subsystem
  Subsystem4 : Subsystem
  rd_dout : Outport  PortDimensions=8  VectorParamsAs1DForOutWhenUnconnected=off
  wires:
  Selector1/1 -> Subsystem1/1(data2)
  Selector/1 -> Subsystem4/1(data2)
  data1/1 -> Selector/1, Selector1/1
  Subsystem1/1(rd_dout1) -> Mux/2
  Subsystem4/1(rd_dout1) -> Mux/1
  Mux/1 -> rd_dout/1
  wr_en1/1 -> Subsystem1/3(wr_en2), Subsystem4/3(wr_en2)
  rd_addr/1 -> Subsystem1/4(rd_addr1), Subsystem4/4(rd_addr1)
  wr_addr/1 -> Subsystem1/2(wr_addr1), Subsystem4/2(wr_addr1)
